simulink model "COMMUNICATION"  (R2023b)
settings: Solver=VariableStepAuto  StartTime=0.0  StopTime=10.0  RelTol=1e-3
settings Model: Creator=lucaerviati  LastModifiedBy=carol
settings DataIOCC: SaveOutput=off  SaveTime=off
settings OptimizationCC: ReuseModelBlockBuffer=off
settings GRTTargetCC: CombineOutputUpdateFcns=off  MatFileLogging=off

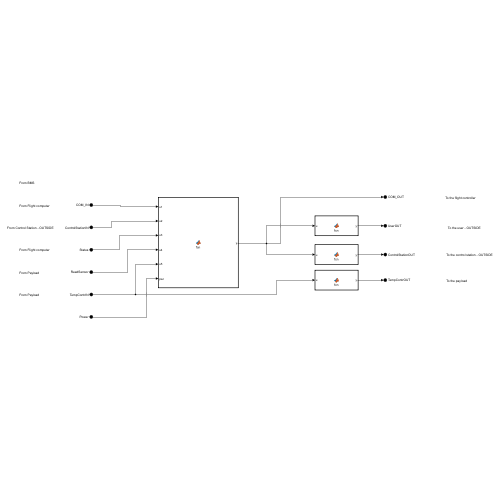
[thumbnail: Simulink's stored preview of the top-level diagram]
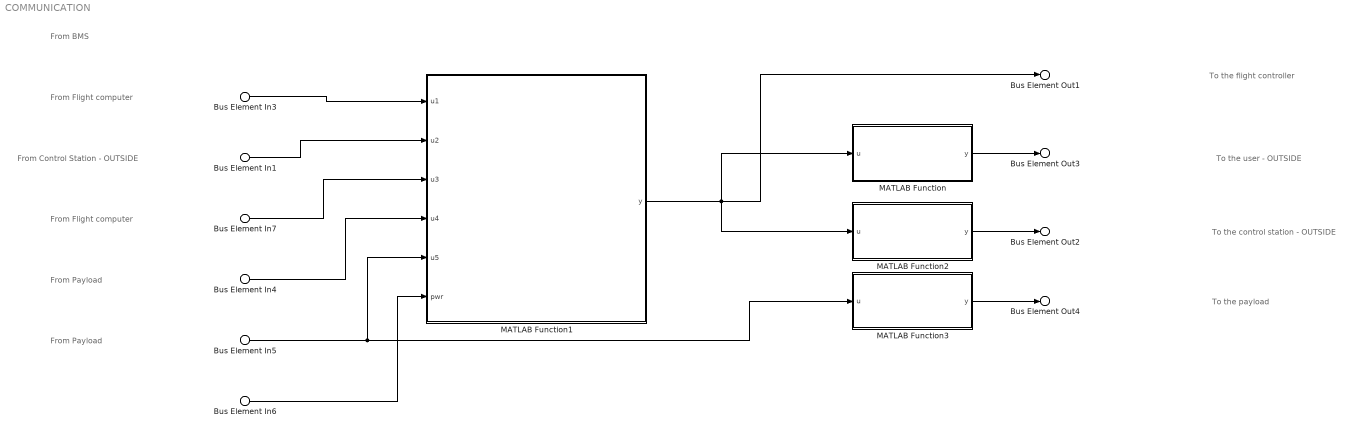
== system COMMUNICATION ==
  note: To the control station - OUTSIDE
  note: To the payload
  note: To the user - OUTSIDE
  note: To the flight controller
  note: From Flight computer
  note: From Control Station - OUTSIDE
  note: From Flight computer
  note: From Payload
  note: From Payload
  note: From BMS
  Bus Element In6 : Inport  PortName=Power
  Bus Element In3 : Inport  Port=2  PortName=COM_IN
  Bus Element In1 : Inport  Port=3  PortName=ControlStationIN
  Bus Element In7 : Inport  Port=4  PortName=Status
  Bus Element In4 : Inport  Port=5  PortName=ReadSensor
  Bus Element In5 : Inport  Port=6  PortName=TempContrIN
  MATLAB Function : MATLAB Function  TreatAsAtomicUnit=on
  MATLAB Function1 : MATLAB Function  TreatAsAtomicUnit=on
  MATLAB Function2 : MATLAB Function  TreatAsAtomicUnit=on
  MATLAB Function3 : MATLAB Function  TreatAsAtomicUnit=on
  Bus Element Out1 : Outport  PortName=COM_OUT
  Bus Element Out3 : Outport  Port=2  PortName=UserOUT
  Bus Element Out2 : Outport  Port=3  PortName=ControlStationOUT
  Bus Element Out4 : Outport  Port=4  PortName=TempContrOUT
  wires:
  MATLAB Function1/1(y) -> MATLAB Function/1(u), MATLAB Function2/1(u), Bus Element Out1/1
  Bus Element In6/1 -> MATLAB Function1/6(pwr)
  Bus Element In3/1 -> MATLAB Function1/1(u1)
  Bus Element In1/1 -> MATLAB Function1/2(u2)
  Bus Element In7/1 -> MATLAB Function1/3(u3)
  Bus Element In4/1 -> MATLAB Function1/4(u4)
  Bus Element In5/1 -> MATLAB Function3/1(u), MATLAB Function1/5(u5)
  MATLAB Function/1(y) -> Bus Element Out3/1
  MATLAB Function2/1(y) -> Bus Element Out2/1
  MATLAB Function3/1(y) -> Bus Element Out4/1

== matlab function COMMUNICATION/MATLAB Function1 ==
  data: u1 input; y output; u2 input; u3 input; u4 input; u5 input; pwr input
function y = fcn(u1,u2,u3,u4,u5, pwr)

u = [1,1,1,1,1,0]




y = u;

== matlab function COMMUNICATION/MATLAB Function ==
  data: u input; y output
function y = fcn(u)
u = 1;
y = u;

== matlab function COMMUNICATION/MATLAB Function2 ==
  data: u input; y output
function y = fcn(u)
u = 1;
y = u;

== matlab function COMMUNICATION/MATLAB Function3 ==
  data: u input; y output
function y = fcn(u)
u = 1;
y = u;
